simulink model "PendulumRCS_Rewrite1"  (R2018b)
settings: Solver=VariableStepAuto  StartTime=0.0  StopTime=6  RelTol=1e-9
model workspace (MAT data in the model file):
  H = 0.4
  I = [32.11828  0  0; 0  32.11828  0; 0  0  0.023226]
  L = 2
  M = 1
  R = 0.0762
libraries: dspmtrx3 x2, sharedutil x1, shared6dof x1, aerolibanim x1, vrlib x1
settings Model: Creator=mendicantbias  LastModifiedBy=mendicantbias

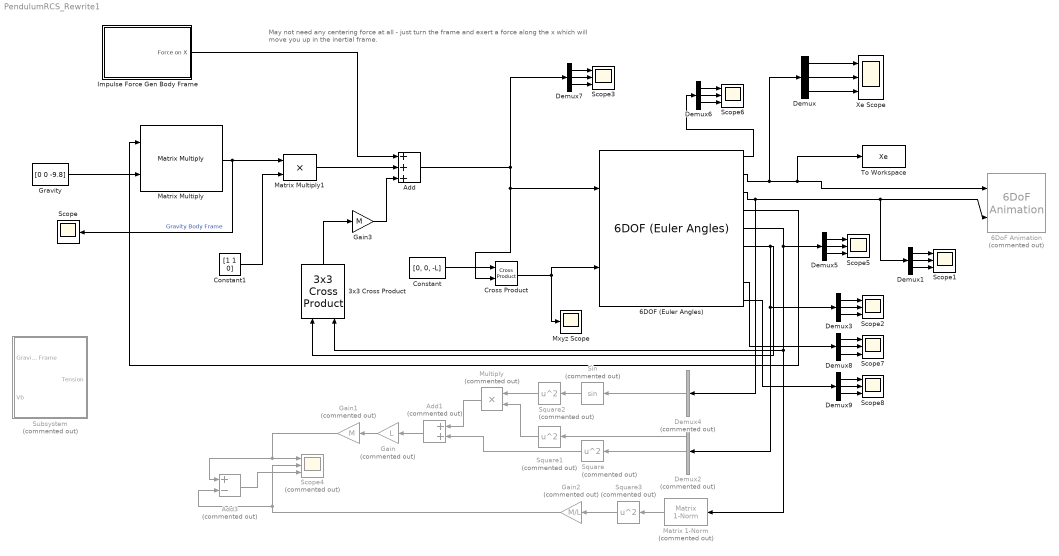
== system PendulumRCS_Rewrite1 ==
  note: May not need any centering force at all - just turn the frame and exert a force along the x which will move you up in the inertial frame.
  3x3 Cross Product : sharedutil/3x3 Cross Product  aMode=aMode
      settings: SourceProductBaseCode=AE
  6DOF (Euler Angles) : shared6dof/6DOF (Euler Angles)  units=Metric (MKS)  mtype=Fixed  rep=Euler Angles  xme_0=[0 0 -L]  Vm_0=[0 0 0]  eul_0=[0 0 0]  pm_0=[0 0 0]  mass_0=1  mass_e=0.5  mass_f=2.0  inertia=eye(3)  inertia_e=eye(3)  inertia_f=2*eye(3)  k_quat=1.0  vre_flag=on  abi_flag=on  aMode=0  xme_statename=''  Vm_statename=''  eul_statename=''  quat_statename=''  pm_statename=''  mass_statename=''
      settings: SourceProductBaseCode=AE
  6DoF Animation : aerolibanim/6DoF Animation  Commented=on  u1=[-5 5 -5 5 -5 5]  u2=0.01  u3=0.2  u4=[4000 0 -5000]  u5=Fly alongside  u6=[-5 -5 5]  u7=30  u8=on
      settings: SourceProductName=Aerospace Blockset
  Add : Sum  Inputs=+++
  Add1 : Sum  Commented=on  Inputs=2
  Add3 : Sum  Commented=on  Inputs=+-
  Constant : Constant  Value=[0, 0, -L]
  Constant1 : Constant  Value=[1 1 0]
  Cross Product : vrlib/Utilities/Cross Product
      settings: SourceProductBaseCode=VR
  Demux{,1,3,5..9} (8 alike) : Demux  Outputs=3
  Demux2 : Demux  Commented=on  Outputs=3
  Demux4 : Demux  Commented=on  Outputs=3
  Gain : Gain  Commented=on  Gain=L
  Gain1 : Gain  Commented=on  Gain=M
  Gain2 : Gain  Commented=on  Gain=M/L
  Gain3 : Gain  Gain=M
  Gravity : Constant  Value=[0 0 -9.8]
  Impulse Force Gen Body Frame : Subsystem
  Matrix 1-Norm : dspmtrx3/Matrix  1-Norm  Commented=on  roundingMode=Floor  overflowMode=off  outputDataTypeStr=Inherit: Same as accumulator  outputMin=[]  outputMax=[]  outputLastDataTypeStr=Inherit: Same as accumulator
      settings: SourceProductName=DSP System Toolbox  SourceProductBaseCode=DS
  Matrix Multiply : Product  Multiplication=Matrix(*)
  Matrix Multiply1 : Product
  Multiply : Product  Commented=on
  Mxyz Scope : Scope
  Scope : Scope
  Scope{1..3,5..8} (7 alike) : Scope  NumInputPorts=3
  Scope4 : Scope  Commented=on  NumInputPorts=3
  Sin : Trigonometry  Commented=on
  Square{,1..3} (4 alike) : Math  Commented=on  Operator=square  SaturateOnIntegerOverflow=on
  Subsystem : Subsystem  Commented=on
  To Workspace : ToWorkspace  VariableName=Xe  SaveFormat=Timeseries  SampleTime=-1
  Xe Scope : Scope  NumInputPorts=3
  wires:
  Matrix Multiply/1 -> Matrix Multiply1/1, Scope/1  "Gravity Body Frame"
  6DOF (Euler Angles)/2 -> Demux/1, 6DoF Animation/1, To Workspace/1
  6DOF (Euler Angles)/3 -> Demux4/1, Demux1/1, 6DoF Animation/2
  Gravity/1 -> Matrix Multiply/2
  6DOF (Euler Angles)/4 -> Matrix Multiply/1
  Add/1 -> Demux7/1, 6DOF (Euler Angles)/1, Cross Product/2
  Demux/3 -> Xe Scope/3
  Demux/2 -> Xe Scope/2
  Demux/1 -> Xe Scope/1
  Constant/1 -> Cross Product/1
  Cross Product/1 -> 6DOF (Euler Angles)/2, Mxyz Scope/1
  Demux1/3 -> Scope1/3
  Demux1/2 -> Scope1/2
  Demux1/1 -> Scope1/1
  Demux3/3 -> Scope2/3
  Demux3/2 -> Scope2/2
  Demux3/1 -> Scope2/1
  6DOF (Euler Angles)/6 -> 3x3 Cross Product/1, Demux2/1, Demux3/1
  Demux2/2 -> Square/1
  Demux2/1 -> Square1/1
  Demux4/2 -> Sin/1
  Sin/1 -> Square2/1
  Square2/1 -> Multiply/1
  Square1/1 -> Multiply/2
  Square/1 -> Add1/2
  Multiply/1 -> Add1/1
  Add1/1 -> Gain/1
  Gain/1 -> Gain1/1
  Gain1/1 -> Add3/1, Scope4/1
  Matrix 1-Norm/1 -> Square3/1
  Square3/1 -> Gain2/1
  6DOF (Euler Angles)/5 -> 3x3 Cross Product/2, Matrix 1-Norm/1, Demux5/1
  Gain2/1 -> Scope4/2, Add3/2
  Add3/1 -> Scope4/3
  Constant1/1 -> Matrix Multiply1/2
  Demux5/2 -> Scope5/2
  Demux5/3 -> Scope5/3
  Demux5/1 -> Scope5/1
  Demux6/2 -> Scope6/2
  Demux6/1 -> Scope6/1
  Demux6/3 -> Scope6/3
  6DOF (Euler Angles)/1 -> Demux6/1
  Matrix Multiply1/1 -> Add/2
  Impulse Force Gen Body Frame/1(Force on X) -> Add/1
  Demux7/3 -> Scope3/3
  Demux7/2 -> Scope3/2
  Demux7/1 -> Scope3/1
  Demux8/3 -> Scope7/3
  Demux8/2 -> Scope7/2
  Demux8/1 -> Scope7/1
  Demux9/3 -> Scope8/3
  Demux9/2 -> Scope8/2
  Demux9/1 -> Scope8/1
  6DOF (Euler Angles)/8 -> Demux8/1
  6DOF (Euler Angles)/9 -> Demux9/1
  3x3 Cross Product/1 -> Gain3/1
  Gain3/1 -> Add/3

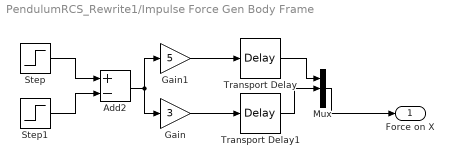
== system PendulumRCS_Rewrite1/Impulse Force Gen Body Frame ==
  Add2 : Sum  Inputs=+-
  Gain : Gain  Gain=3
  Gain1 : Gain  Gain=5
  Mux : Mux  Inputs=3
  Step : Step  SampleTime=0
  Step1 : Step  Time=1.5  SampleTime=0
  Transport Delay : TransportDelay  DelayTime=0
  Transport Delay1 : TransportDelay  DelayTime=0.3
  Force on X : Outport
  wires:
  Step/1 -> Add2/1
  Step1/1 -> Add2/2
  Add2/1 -> Gain/1, Gain1/1
  Gain1/1 -> Transport Delay/1
  Mux/1 -> Force on X/1
  Gain/1 -> Transport Delay1/1
  Transport Delay/1 -> Mux/1
  Transport Delay1/1 -> Mux/2

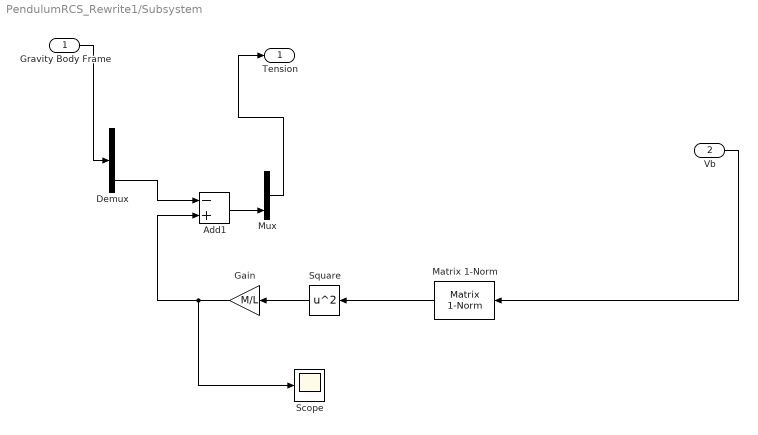
== system PendulumRCS_Rewrite1/Subsystem ==
  Gravity Body Frame : Inport
  Vb : Inport  Port=2
  Add1 : Sum  Inputs=-+
  Demux : Demux  Outputs=3
  Gain : Gain  Gain=M/L
  Matrix 1-Norm : dspmtrx3/Matrix  1-Norm  roundingMode=Floor  overflowMode=off  outputDataTypeStr=Inherit: Same as accumulator  outputMin=[]  outputMax=[]  outputLastDataTypeStr=Inherit: Same as accumulator
      settings: SourceProductName=DSP System Toolbox  SourceProductBaseCode=DS
  Mux : Mux  Inputs=3
  Scope : Scope
  Square : Math  Operator=square  SaturateOnIntegerOverflow=on
  Tension : Outport
  wires:
  Add1/1 -> Mux/3
  Gain/1 -> Scope/1, Add1/2
  Matrix 1-Norm/1 -> Square/1
  Gravity Body Frame/1 -> Demux/1
  Mux/1 -> Tension/1
  Square/1 -> Gain/1
  Demux/3 -> Add1/1
  Vb/1 -> Matrix 1-Norm/1
